simulink model "speedgoat_target_model_2021b"  (R2021b)
settings: Solver=FixedStepAuto  StartTime=0.0  StopTime=inf  RelTol=1e-3
undefined symbols (not defined in the file): DEND_B, DEND_T, DiscIntNeverNeededParam, NUMD_B, NUMD_T, ts
libraries: slrealtimeutilitieslib x7, slrealtimeiplib x7, simulink x5, drivingvehiclecontroller x2, mpcadaslib x1
settings Model: Creator=Buckeye Autodrive  LastModifiedBy=Buckeye Autodrive
settings SolverCC: ConcurrentTasks=on  PositivePriorityOrder=on  AutoInsertRateTranBlk=on
settings OptimizationCC: BlockReduction=off  OptimizeBlockIOStorage=off
settings DebuggingCC: TasksWithSamePriorityMsg=none  UnconnectedInputMsg=none  UnconnectedOutputMsg=none  UnconnectedLineMsg=none
settings HardwareCC: ProdBitPerLong=64  ProdLongLongMode=on  ProdHWDeviceType=Intel->x86-64 (Linux 64)
settings ModelReferenceCC: EnableRefExpFcnMdlSchedulingChecks=off
settings RTWCC: Description=Simulink Real-Time  SystemTargetFile=slrealtime.tlc  TemplateMakefile=slrealtime_default_tmf  Toolchain=Simulink Real-Time Toolchain  BuildConfiguration=Faster Runs  CodeExecutionProfiling=on  TargetLang=C++  DLArmComputeVersion=20.02.1

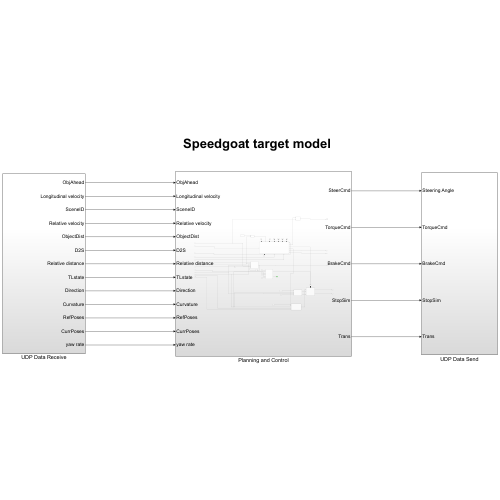
[thumbnail: Simulink's stored preview of the top-level diagram]
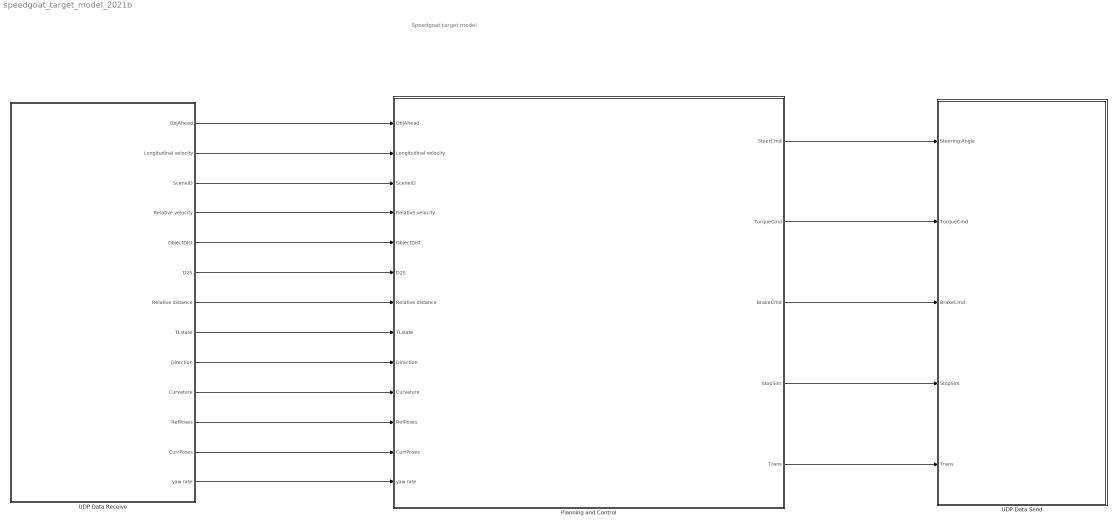
== system speedgoat_target_model_2021b ==
  note: Speedgoat target model
  Planning and Control : Subsystem
  UDP Data Receive : Subsystem
  UDP Data Send : Subsystem
  wires:
  Planning and Control/1(SteerCmd) -> UDP Data Send/1(Steering Angle)
  Planning and Control/2(TorqueCmd) -> UDP Data Send/2(TorqueCmd)
  Planning and Control/3(BrakeCmd) -> UDP Data Send/3(BrakeCmd)
  Planning and Control/4(StopSim) -> UDP Data Send/4(StopSim)
  Planning and Control/5(Trans) -> UDP Data Send/5(Trans)
  UDP Data Receive/1(ObjAhead) -> Planning and Control/1(ObjAhead)
  UDP Data Receive/2(Longitudinal velocity) -> Planning and Control/2(Longitudinal velocity)
  UDP Data Receive/3(SceneID) -> Planning and Control/3(SceneID)
  UDP Data Receive/4(Relative velocity) -> Planning and Control/4(Relative velocity)
  UDP Data Receive/5(ObjectDist) -> Planning and Control/5(ObjectDist)
  UDP Data Receive/6(D2S) -> Planning and Control/6(D2S)
  UDP Data Receive/7(Relative distance) -> Planning and Control/7(Relative distance)
  UDP Data Receive/8(TLstate) -> Planning and Control/8(TLstate)
  UDP Data Receive/9(Direction) -> Planning and Control/9(Direction)
  UDP Data Receive/10(Curvature) -> Planning and Control/10(Curvature)
  UDP Data Receive/11(RefPoses) -> Planning and Control/11(RefPoses)
  UDP Data Receive/12(CurrPoses) -> Planning and Control/12(CurrPoses)
  UDP Data Receive/13(yaw rate) -> Planning and Control/13(yaw rate)

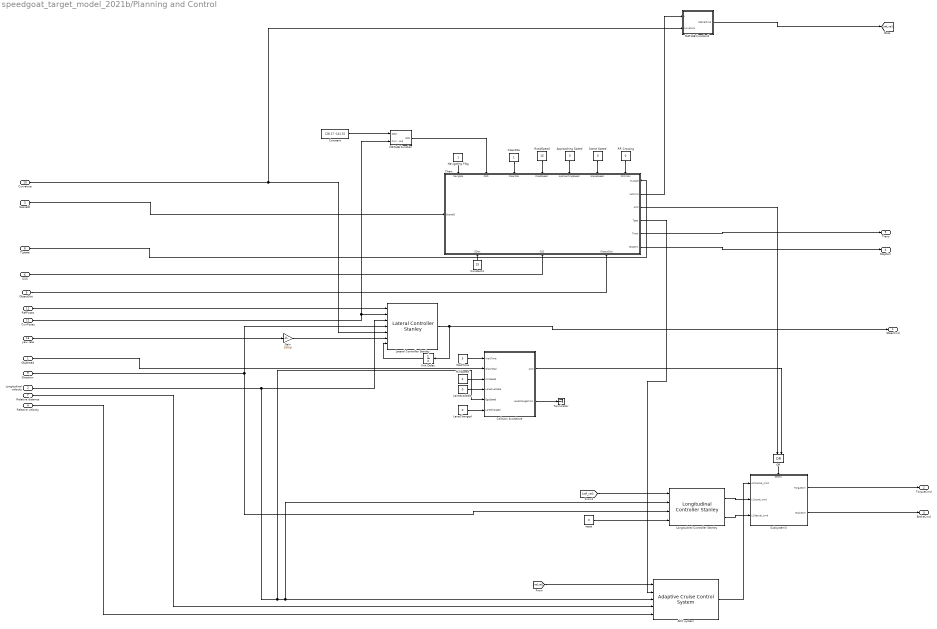
== system speedgoat_target_model_2021b/Planning and Control ==
  ObjAhead : Inport
  Longitudinal velocity : Inport  Port=2
  SceneID : Inport  Port=3
  Relative velocity : Inport  Port=4
  ObjectDist : Inport  Port=5
  D2S : Inport  Port=6
  Relative distance : Inport  Port=7
  TLstate : Inport  Port=8
  Direction : Inport  Port=9
  Curvature : Inport  Port=10
  RefPoses : Inport  Port=11
  CurrPoses : Inport  Port=12
  yaw rate : Inport  Port=13
  ACC system : mpcadaslib/Adaptive Cruise Control System  EgoModel=tf(1,[0.5,1,0])  InitialEgoVelocity=0  DefaultSpacing=4.685  MaxVelocity=50  MinAcceleration=-40  amin_ext=off  MaxAcceleration=40  amax_ext=off  Ts=1  PredictionHorizon=10  ControllerBehavior=1.0  suboptimal=off  maxiter=10  datatypeopt=double  optmode=off  trackmode=off
  Approaching Speed : Constant  Value=5
  Chart : Stateflow chart  TreatAsAtomicUnit=on
      settings: PortSchema="{\"entries\":[{\"content\":{\"sides\":[{\"content\":{\"connectorIds\":[\"In12\"]},\"type\":\"ConnectorPlacement.EquallySpacedRectSide\",\"uuid\":\"81aca70f-0947-49fb-b60a-be241e44193b\"},{\"content\":{\"connectorIds\":[\"In1\",\"Out1\",\"Out2\",\"Out3\",\"Out4\",\"Out5\"],\"side\":\"RIGHT\"},\"type\":\"ConnectorPlacement.EquallySpacedRectSide\",\"uuid\":\"e7b9645e-3711-4964-ac9b-0199dd335e99\"},{\"content\":{\"connectorIds\":[\"In8\",\"In9\",\"In10\",\"In11\",\"In2\",\"In4\",\"In6\"],\"side\":\"TOP\"},\"type\":\"ConnectorPlacement.EquallySpacedRectSide\",\"uuid\":\"6876f024-944b-4540-9404-d68f37763657\"},{\"content\":{\"connectorIds\":[\"In5\",\"In7\",\"In3\"],\"side\":\"BOTTOM\"},\"type\":\"ConnectorPlacement.EquallySpacedRectSide\",\"uuid\":\"44acab73-cdde-4edf-95df-27422644ccab\"}]},\"type\":\"ConnectorPlacement.EquallySpacedConnector\",\"uuid\":\"d2c31c01-e447-43db-8d2b-8b98a0ca291a\"}],\"packageUris\":[\"http://schema.mathworks.com/mf0/Connector/R2020b\"],\"version\":\"1.0\"}"
  Clear2Go : Constant
  Collision Avoidance : Stateflow chart  TreatAsAtomicUnit=on
  Constant : Constant  Value=[28.17 -141.5]
  Constant1 : Constant  Value=25
  Gain : Gain  Gain=180/pi
  LaneAvailable : Constant  Value=0
  LaneChanged : Constant  Value=0
  Lateral Controller Stanley : drivingvehiclecontroller/Lateral Controller Stanley  ModelType=Dynamic bicycle model  PositionGainF=2.5  PositionGainR=2.5  YawRateGain=0.2  DelayGain=0.2  VehicleMass=1853  Lf=1.3425  Lr=1.3425  TireStiffness=5e3  Wheelbase=3  MaxSteeringAngle=80
      settings: SourceProductBaseCode=DR
  Longitudinal Controller Stanley : drivingvehiclecontroller/Longitudinal Controller Stanley  Kp=10  Ki=0.1  SampleTime=1  MaxAcceleration=40  MaxDeceleration=40
      settings: SourceProductBaseCode=DR
  MATLAB Function : MATLAB Function  TreatAsAtomicUnit=on
  MATLAB Function2 : MATLAB Function  TreatAsAtomicUnit=on
  MinSpeed : Constant  Value=2
  Navigating Flag : Constant
  OR : Logic  Operator=OR  IconShape=distinctive  AllPortsSameDT=off  OutDataTypeStr=fixdt(1,16)
  RR Crossing : Constant  Value=0
  RoadSpeed : Constant  Value=15
  Scene Speed : Constant  Value=5
  Subsystem3 : Subsystem
      settings: PortSchema="{\"entries\":[{\"content\":{\"sides\":[{\"content\":{\"connectorIds\":[\"In1\",\"In2\",\"In3\"]},\"type\":\"ConnectorPlacement.EquallySpacedRectSide\",\"uuid\":\"a23b1a10-3bcb-40a0-900c-c9a3f160b173\"},{\"content\":{\"connectorIds\":[\"Out1\",\"Out2\"],\"side\":\"RIGHT\"},\"type\":\"ConnectorPlacement.EquallySpacedRectSide\",\"uuid\":\"88840b66-912f-4184-aeec-297642319416\"},{\"content\":{\"connectorIds\":[\"In4\"],\"side\":\"TOP\"},\"type\":\"ConnectorPlacement.EquallySpacedRectSide\",\"uuid\":\"37a03ca9-b065-473e-b290-3b07703c6005\"}]},\"type\":\"ConnectorPlacement.EquallySpacedConnector\",\"uuid\":\"5bfc7c71-8f7a-4cba-a168-7eeca22a2fcb\"}],\"packageUris\":[\"http://schema.mathworks.com/mf0/Connector/R2020b\"],\"version\":\"1.0\"}"
  Terminator : Terminator
  Unit Delay : UnitDelay  SampleTime=-1  HasFrameUpgradeWarning=on
  WaitTime : Constant  Value=3
  reset : Constant  Value=0
  SteerCmd : Outport
  TorqueCmd : Outport  Port=2
  BrakeCmd : Outport  Port=3
  StopSim : Outport  Port=4
  Trans : Outport  Port=5
  wires:
  TLstate/1 -> Chart/1(TLstate)
  Chart/3(Tgap) -> ACC system/2
  Collision Avoidance/2(LaneChangeCmd) -> Terminator/1
  Navigating Flag/1 -> Chart/8(Navigate)
  Longitudinal velocity/1 -> Collision Avoidance/5(EgoSpeed), Longitudinal Controller Stanley/2, ACC system/3, Lateral Controller Stanley/3
  MinSpeed/1 -> Collision Avoidance/3(MinSpeed)
  RefPoses/1 -> Lateral Controller Stanley/1
  yaw rate/1 -> Gain/1
  Lateral Controller Stanley/1 -> Unit Delay/1, SteerCmd/1
  Constant1/1 -> Chart/5(SDist)
  ACC system/1 -> Subsystem3/1(ACCaccel_cmd)
  Scene Speed/1 -> Chart/4(SceneSpeed)
  Curvature/1 -> Lateral Controller Stanley/5, MATLAB Function2/2(curvature)
  Chart/2(ACC) -> OR/1
  [ref_vel] -> ACC system/1
  Collision Avoidance/1(ACC) -> OR/2
  [ref_vel] -> Longitudinal Controller Stanley/1
  Subsystem3/1(TorgueCm) -> TorqueCmd/1
  ObjAhead/1 -> Collision Avoidance/2(ObjAhead)
  SceneID/1 -> Chart/12(SceneID)
  Direction/1 -> Longitudinal Controller Stanley/3, Lateral Controller Stanley/4
  MATLAB Function/1(D2D) -> Chart/9(D2D)
  Constant/1 -> MATLAB Function/1(Dest)
  RoadSpeed/1 -> Chart/11(RoadSpeed)
  Longitudinal Controller Stanley/1 -> Subsystem3/2(LCaccel_cmd)
  reset/1 -> Longitudinal Controller Stanley/4
  CurrPoses/1 -> MATLAB Function/2(CurrentPose), Lateral Controller Stanley/2
  LaneChanged/1 -> Collision Avoidance/6(LaneChanged)
  Clear2Go/1 -> Chart/10(Clear2Go)
  Longitudinal Controller Stanley/2 -> Subsystem3/3(LCdeccel_cmd)
  RR Crossing/1 -> Chart/6(RRCross)
  Chart/1(VelCmd) -> MATLAB Function2/1(v)
  ObjectDist/1 -> Chart/3(ObjectDist)
  WaitTime/1 -> Collision Avoidance/1(WaitTime)
  Chart/4(Trans) -> Trans/1
  LaneAvailable/1 -> Collision Avoidance/4(LaneAvailable)
  Chart/5(StopSim) -> StopSim/1
  Approaching Speed/1 -> Chart/2(ApproachingSpeed)
  OR/1 -> Subsystem3/4(Select)
  Relative distance/1 -> ACC system/4
  Subsystem3/2(BrakeCm) -> BrakeCmd/1
  Relative velocity/1 -> ACC system/5
  D2S/1 -> Chart/7(D2S)
  MATLAB Function2/1(RefVelCmd) -> [ref_vel]
  Gain/1 -> Lateral Controller Stanley/6
  Unit Delay/1 -> Lateral Controller Stanley/7

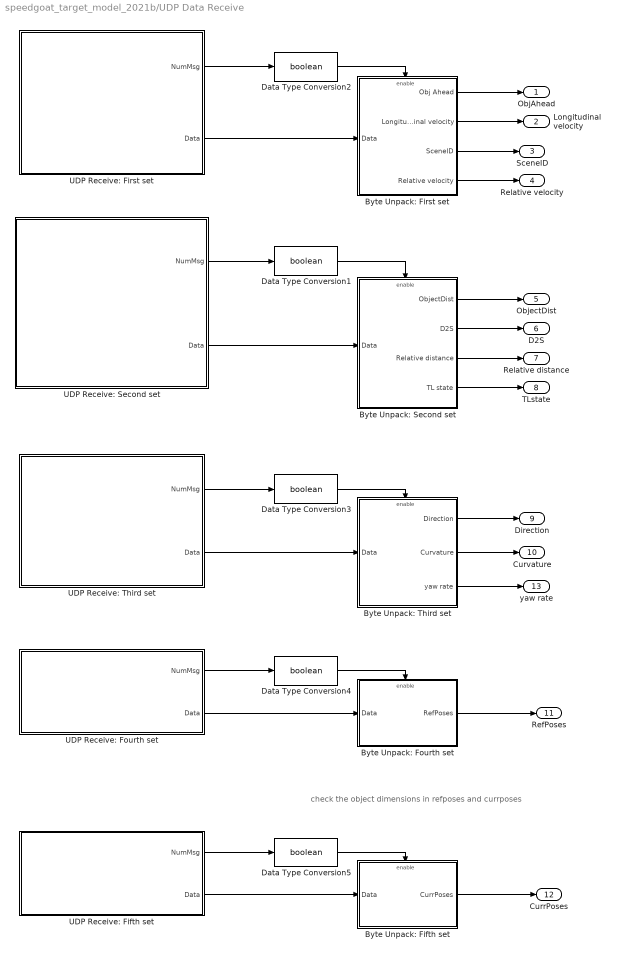
== system speedgoat_target_model_2021b/UDP Data Receive ==
  note: check the object dimensions in refposes and currposes
  Byte Unpack: Fifth set : Subsystem
  Byte Unpack: First set : Subsystem
  Byte Unpack: Fourth set : Subsystem
  Byte Unpack: Second set : Subsystem
  Byte Unpack: Third set : Subsystem
  Data Type Conversion{1..5} (5 alike) : DataTypeConversion  OutDataTypeStr=boolean
  UDP Receive: Fifth set : Subsystem
  UDP Receive: First set : Subsystem
  UDP Receive: Fourth set : Subsystem
  UDP Receive: Second set : Subsystem
  UDP Receive: Third set : Subsystem
  ObjAhead : Outport
  Longitudinal velocity : Outport  Port=2
  SceneID : Outport  Port=3
  Relative velocity : Outport  Port=4
  ObjectDist : Outport  Port=5
  D2S : Outport  Port=6
  Relative distance : Outport  Port=7
  TLstate : Outport  Port=8
  Direction : Outport  Port=9
  Curvature : Outport  Port=10
  RefPoses : Outport  Port=11
  CurrPoses : Outport  Port=12
  yaw rate : Outport  Port=13
  wires:
  UDP Receive: First set/1(NumMsg) -> Data Type Conversion2/1
  Data Type Conversion2/1 -> Byte Unpack: First set/Enable
  UDP Receive: First set/2(Data) -> Byte Unpack: First set/1(Data)
  UDP Receive: Second set/2(Data) -> Byte Unpack: Second set/1(Data)
  Data Type Conversion1/1 -> Byte Unpack: Second set/Enable
  UDP Receive: Second set/1(NumMsg) -> Data Type Conversion1/1
  UDP Receive: Third set/1(NumMsg) -> Data Type Conversion3/1
  Data Type Conversion3/1 -> Byte Unpack: Third set/Enable
  UDP Receive: Third set/2(Data) -> Byte Unpack: Third set/1(Data)
  UDP Receive: Fifth set/2(Data) -> Byte Unpack: Fifth set/1(Data)
  Data Type Conversion5/1 -> Byte Unpack: Fifth set/Enable
  UDP Receive: Fifth set/1(NumMsg) -> Data Type Conversion5/1
  UDP Receive: Fourth set/1(NumMsg) -> Data Type Conversion4/1
  Data Type Conversion4/1 -> Byte Unpack: Fourth set/Enable
  UDP Receive: Fourth set/2(Data) -> Byte Unpack: Fourth set/1(Data)
  Byte Unpack: First set/1(Obj Ahead) -> ObjAhead/1
  Byte Unpack: First set/2(Longitudinal velocity) -> Longitudinal velocity/1
  Byte Unpack: First set/3(SceneID) -> SceneID/1
  Byte Unpack: First set/4(Relative velocity) -> Relative velocity/1
  Byte Unpack: Second set/1(ObjectDist) -> ObjectDist/1
  Byte Unpack: Second set/2(D2S) -> D2S/1
  Byte Unpack: Second set/3(Relative distance) -> Relative distance/1
  Byte Unpack: Second set/4(TL state) -> TLstate/1
  Byte Unpack: Fourth set/1(RefPoses) -> RefPoses/1
  Byte Unpack: Fifth set/1(CurrPoses) -> CurrPoses/1
  Byte Unpack: Third set/1(Direction) -> Direction/1
  Byte Unpack: Third set/2(Curvature) -> Curvature/1
  Byte Unpack: Third set/3(yaw rate) -> yaw rate/1

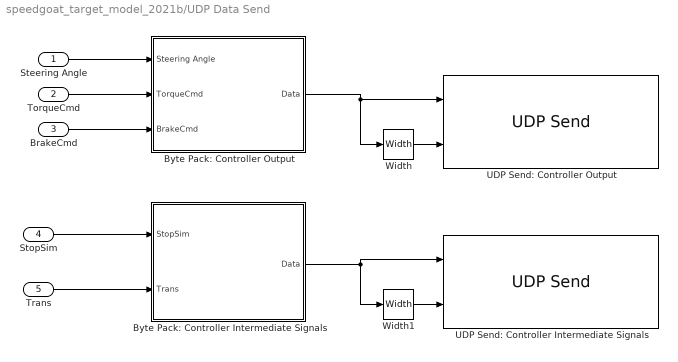
== system speedgoat_target_model_2021b/UDP Data Send ==
  Steering Angle : Inport
  TorqueCmd : Inport  Port=2
  BrakeCmd : Inport  Port=3
  StopSim : Inport  Port=4
  Trans : Inport  Port=5
  Byte Pack: Controller Intermediate Signals : Subsystem
  Byte Pack: Controller Output : Subsystem
  UDP Send: Controller Intermediate Signals : slrealtimeiplib/UDP Send  useHostTargetConn=on  toAddress=192.168.7.1  toPort=8017  sampleTime=0.1  ipAddress=192.168.7.2  localPort=-1
      settings: SourceProductBaseCode=XP
  UDP Send: Controller Output : slrealtimeiplib/UDP Send  useHostTargetConn=on  toAddress=192.168.7.1  toPort=8016  sampleTime=0.1  ipAddress=192.168.7.2  localPort=-1
      settings: SourceProductBaseCode=XP
  Width : Width
  Width1 : Width
  wires:
  Width1/1 -> UDP Send: Controller Intermediate Signals/2
  Width/1 -> UDP Send: Controller Output/2
  Byte Pack: Controller Output/1(Data) -> Width/1, UDP Send: Controller Output/1
  Steering Angle/1 -> Byte Pack: Controller Output/1(Steering Angle)
  TorqueCmd/1 -> Byte Pack: Controller Output/2(TorqueCmd)
  Byte Pack: Controller Intermediate Signals/1(Data) -> UDP Send: Controller Intermediate Signals/1, Width1/1
  StopSim/1 -> Byte Pack: Controller Intermediate Signals/1(StopSim)
  Trans/1 -> Byte Pack: Controller Intermediate Signals/2(Trans)
  BrakeCmd/1 -> Byte Pack: Controller Output/3(BrakeCmd)

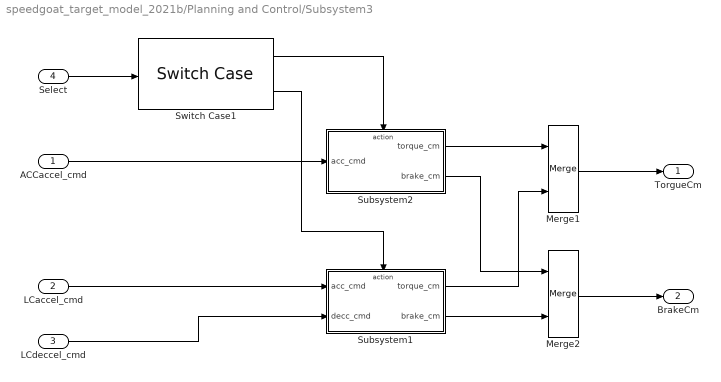
== system speedgoat_target_model_2021b/Planning and Control/Subsystem3 ==
  ACCaccel_cmd : Inport
  LCaccel_cmd : Inport  Port=2
  LCdeccel_cmd : Inport  Port=3
  Select : Inport  Port=4
  Merge1 : Merge
  Merge2 : Merge
  Subsystem1 : Subsystem
  Subsystem2 : Subsystem
  Switch Case1 : SwitchCase  CaseConditions={1, 0}  ShowDefaultCase=off
  TorgueCm : Outport
  BrakeCm : Outport  Port=2
  wires:
  LCdeccel_cmd/1 -> Subsystem1/2(decc_cmd)
  Subsystem1/2(brake_cm) -> Merge2/2
  Subsystem1/1(torque_cm) -> Merge1/2
  Subsystem2/2(brake_cm) -> Merge2/1
  Switch Case1/1 -> Subsystem2/Action
  Switch Case1/2 -> Subsystem1/Action
  Subsystem2/1(torque_cm) -> Merge1/1
  LCaccel_cmd/1 -> Subsystem1/1(acc_cmd)
  Merge2/1 -> BrakeCm/1
  ACCaccel_cmd/1 -> Subsystem2/1(acc_cmd)
  Merge1/1 -> TorgueCm/1
  Select/1 -> Switch Case1/1

== system speedgoat_target_model_2021b/UDP Data Receive/Byte Unpack: Fifth set ==
  Data : Inport
  Enable : EnablePort
  Byte Unpacking 1 : slrealtimeutilitieslib/Byte Unpacking  MaskUnpackedDataTypes={'double'}  MaskUnpackedDataSizes={[3]}  MaskAlignment=1
      settings: SourceProductBaseCode=XP
  CurrPoses : Outport
  wires:
  Data/1 -> Byte Unpacking 1/1
  Byte Unpacking 1/1 -> CurrPoses/1  "CurrPoses"

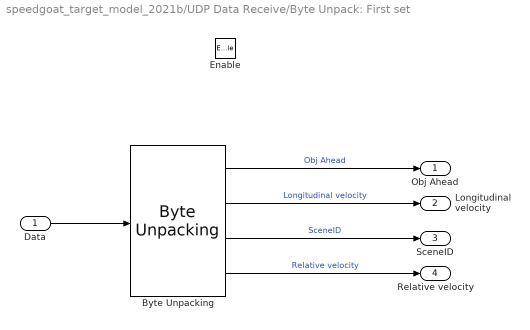
== system speedgoat_target_model_2021b/UDP Data Receive/Byte Unpack: First set ==
  Data : Inport
  Enable : EnablePort
  "Byte Unpacking " : slrealtimeutilitieslib/Byte Unpacking  MaskUnpackedDataTypes={'double', 'double', 'double', 'double'}  MaskUnpackedDataSizes={[1], [1], [1], [1]}  MaskAlignment=1
      settings: SourceProductBaseCode=XP
  Obj Ahead : Outport
  Longitudinal velocity : Outport  Port=2
  SceneID : Outport  Port=3
  Relative velocity : Outport  Port=4
  wires:
  Data/1 -> "Byte Unpacking "/1
  "Byte Unpacking "/1 -> Obj Ahead/1  "Obj Ahead"
  "Byte Unpacking "/2 -> Longitudinal velocity/1  "Longitudinal velocity"
  "Byte Unpacking "/3 -> SceneID/1  "SceneID"
  "Byte Unpacking "/4 -> Relative velocity/1  "Relative velocity"

== system speedgoat_target_model_2021b/UDP Data Receive/Byte Unpack: Fourth set ==
  Data : Inport
  Enable : EnablePort
  "Byte Unpacking " : slrealtimeutilitieslib/Byte Unpacking  MaskUnpackedDataTypes={'double'}  MaskUnpackedDataSizes={[3]}  MaskAlignment=1
      settings: SourceProductBaseCode=XP
  RefPoses : Outport
  wires:
  Data/1 -> "Byte Unpacking "/1
  "Byte Unpacking "/1 -> RefPoses/1  "RefPoses"

== system speedgoat_target_model_2021b/UDP Data Receive/Byte Unpack: Second set ==
  Data : Inport
  Enable : EnablePort
  "Byte Unpacking " : slrealtimeutilitieslib/Byte Unpacking  MaskUnpackedDataTypes={'double', 'double', 'double', 'double'}  MaskUnpackedDataSizes={[1], [1], [1], [18,5]}  MaskAlignment=1
      settings: SourceProductBaseCode=XP
  ObjectDist : Outport
  D2S : Outport  Port=2
  Relative distance : Outport  Port=3
  TL state : Outport  Port=4
  wires:
  "Byte Unpacking "/4 -> TL state/1  "TL state"
  "Byte Unpacking "/3 -> Relative distance/1  "Relative distance"
  "Byte Unpacking "/2 -> D2S/1  "D2S"
  "Byte Unpacking "/1 -> ObjectDist/1  "ObjectDist"
  Data/1 -> "Byte Unpacking "/1

== system speedgoat_target_model_2021b/UDP Data Receive/Byte Unpack: Third set ==
  Data : Inport
  Enable : EnablePort
  "Byte Unpacking " : slrealtimeutilitieslib/Byte Unpacking  MaskUnpackedDataTypes={'double', 'double', 'double'}  MaskUnpackedDataSizes={[1], [1], [1]}  MaskAlignment=1
      settings: SourceProductBaseCode=XP
  Direction : Outport
  Curvature : Outport  Port=2
  yaw rate : Outport  Port=3
  wires:
  Data/1 -> "Byte Unpacking "/1
  "Byte Unpacking "/1 -> Direction/1  "Direction"
  "Byte Unpacking "/2 -> Curvature/1  "Curvature"
  "Byte Unpacking "/3 -> yaw rate/1  "yaw rate"

== system speedgoat_target_model_2021b/UDP Data Receive/UDP Receive: Fifth set ==
  Compare To Constant : simulink/Logic and Bit Operations/Compare To Constant  relop===  const=24  OutDataTypeStr=boolean
  Constant : Constant
  Subtract : Sum  Inputs=+-
  UDP Receive2 : slrealtimeiplib/UDP Receive  useHostTargetConn=on  ipAddress=192.168.7.2  localPort=8005  rcvWidth=24  rcvFmAny=off  fmAddress=192.168.7.1  sampleTime=-1
      settings: SourceProductBaseCode=XP
  While Iterator : WhileIterator  WhileBlockType=do-while  ResetStates=reset  ShowIterationPort=on
  NumMsg : Outport
  Data : Outport  Port=2
  wires:
  While Iterator/1 -> Subtract/1
  UDP Receive2/2 -> Compare To Constant/1
  Subtract/1 -> NumMsg/1
  Constant/1 -> Subtract/2
  UDP Receive2/1 -> Data/1
  Compare To Constant/1 -> While Iterator/1

== system speedgoat_target_model_2021b/UDP Data Receive/UDP Receive: First set ==
  Compare To Constant : simulink/Logic and Bit Operations/Compare To Constant  relop===  const=32  OutDataTypeStr=boolean
  Constant : Constant
  Subtract : Sum  Inputs=+-
  UDP Receive2 : slrealtimeiplib/UDP Receive  useHostTargetConn=on  ipAddress=192.168.7.2  localPort=8001  rcvWidth=32  rcvFmAny=off  fmAddress=192.168.7.1  sampleTime=-1
      settings: SourceProductBaseCode=XP
  While Iterator : WhileIterator  WhileBlockType=do-while  ResetStates=reset  ShowIterationPort=on
  NumMsg : Outport
  Data : Outport  Port=2
  wires:
  Compare To Constant/1 -> While Iterator/1
  UDP Receive2/1 -> Data/1
  Constant/1 -> Subtract/2
  Subtract/1 -> NumMsg/1
  UDP Receive2/2 -> Compare To Constant/1
  While Iterator/1 -> Subtract/1

== system speedgoat_target_model_2021b/UDP Data Receive/UDP Receive: Fourth set ==
  Compare To Constant : simulink/Logic and Bit Operations/Compare To Constant  relop===  const=24  OutDataTypeStr=boolean
  Constant : Constant
  Subtract : Sum  Inputs=+-
  UDP Receive2 : slrealtimeiplib/UDP Receive  useHostTargetConn=on  ipAddress=192.168.7.2  localPort=8004  rcvWidth=24  rcvFmAny=off  fmAddress=192.168.7.1  sampleTime=-1
      settings: SourceProductBaseCode=XP
  While Iterator : WhileIterator  WhileBlockType=do-while  ResetStates=reset  ShowIterationPort=on
  NumMsg : Outport
  Data : Outport  Port=2
  wires:
  Compare To Constant/1 -> While Iterator/1
  UDP Receive2/1 -> Data/1
  Constant/1 -> Subtract/2
  Subtract/1 -> NumMsg/1
  UDP Receive2/2 -> Compare To Constant/1
  While Iterator/1 -> Subtract/1

== system speedgoat_target_model_2021b/UDP Data Receive/UDP Receive: Second set ==
  Compare To Constant : simulink/Logic and Bit Operations/Compare To Constant  relop===  const=744  OutDataTypeStr=boolean
  Constant : Constant
  Subtract : Sum  Inputs=+-
  UDP Receive2 : slrealtimeiplib/UDP Receive  useHostTargetConn=on  ipAddress=192.168.7.2  localPort=8002  rcvWidth=744  rcvFmAny=off  fmAddress=192.168.7.1  sampleTime=-1
      settings: SourceProductBaseCode=XP
  While Iterator : WhileIterator  WhileBlockType=do-while  ResetStates=reset  ShowIterationPort=on
  NumMsg : Outport
  Data : Outport  Port=2
  wires:
  While Iterator/1 -> Subtract/1
  UDP Receive2/2 -> Compare To Constant/1
  Subtract/1 -> NumMsg/1
  Constant/1 -> Subtract/2
  UDP Receive2/1 -> Data/1
  Compare To Constant/1 -> While Iterator/1

== system speedgoat_target_model_2021b/UDP Data Receive/UDP Receive: Third set ==
  Compare To Constant : simulink/Logic and Bit Operations/Compare To Constant  relop===  const=24  OutDataTypeStr=boolean
  Constant : Constant
  Subtract : Sum  Inputs=+-
  UDP Receive2 : slrealtimeiplib/UDP Receive  useHostTargetConn=on  ipAddress=192.168.7.2  localPort=8003  rcvWidth=24  rcvFmAny=off  fmAddress=192.168.7.1  sampleTime=-1
      settings: SourceProductBaseCode=XP
  While Iterator : WhileIterator  WhileBlockType=do-while  ResetStates=reset  ShowIterationPort=on
  NumMsg : Outport
  Data : Outport  Port=2
  wires:
  Compare To Constant/1 -> While Iterator/1
  UDP Receive2/1 -> Data/1
  Constant/1 -> Subtract/2
  Subtract/1 -> NumMsg/1
  UDP Receive2/2 -> Compare To Constant/1
  While Iterator/1 -> Subtract/1

== system speedgoat_target_model_2021b/UDP Data Send/Byte Pack: Controller Intermediate Signals ==
  StopSim : Inport
  Trans : Inport  Port=2
  Byte Packing1 : slrealtimeutilitieslib/Byte Packing  MaskPackedDataType=uint8  MaskUnpackedDataTypes={'double', 'double'}  MaskAlignment=1
  Data : Outport
  wires:
  Byte Packing1/1 -> Data/1
  StopSim/1 -> Byte Packing1/1
  Trans/1 -> Byte Packing1/2

== system speedgoat_target_model_2021b/UDP Data Send/Byte Pack: Controller Output ==
  Steering Angle : Inport
  TorqueCmd : Inport  Port=2
  BrakeCmd : Inport  Port=3
  Byte Packing : slrealtimeutilitieslib/Byte Packing  MaskPackedDataType=uint8  MaskUnpackedDataTypes={'double', 'double','double'}  MaskAlignment=1
  Data : Outport
  wires:
  TorqueCmd/1 -> Byte Packing/2
  Byte Packing/1 -> Data/1
  Steering Angle/1 -> Byte Packing/1
  BrakeCmd/1 -> Byte Packing/3

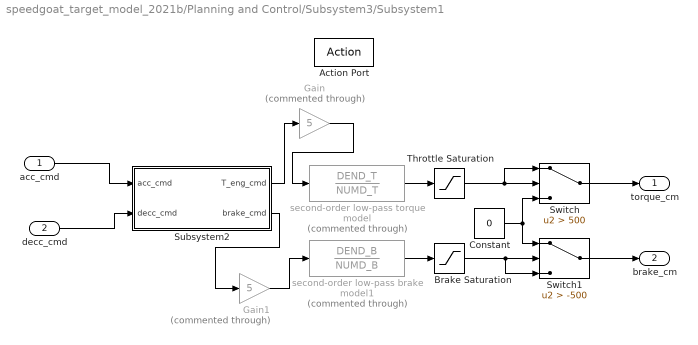
== system speedgoat_target_model_2021b/Planning and Control/Subsystem3/Subsystem1 ==
  acc_cmd : Inport
  decc_cmd : Inport  Port=2
  Action Port : ActionPort  ActionPortLabel=case [ 0 ]:
  Brake Saturation : Saturate  UpperLimit=0  LowerLimit=-65534
  Constant : Constant  Value=0
  Gain : Gain  Commented=through  Gain=5
  Gain1 : Gain  Commented=through  Gain=5
  Subsystem2 : Subsystem
  Switch : Switch  Criteria=u2 > Threshold  Threshold=500
  Switch1 : Switch  Criteria=u2 > Threshold  Threshold=-500
  Throttle Saturation : Saturate  UpperLimit=22534  LowerLimit=-22534
  second-order low-pass brake model1 : DiscreteTransferFcn  Commented=through  Numerator=DEND_B  Denominator=NUMD_B  SampleTime=ts
  second-order low-pass torque model : DiscreteTransferFcn  Commented=through  Numerator=DEND_T  Denominator=NUMD_T  SampleTime=ts
  torque_cm : Outport
  brake_cm : Outport  Port=2
  wires:
  acc_cmd/1 -> Subsystem2/1(acc_cmd)
  Throttle Saturation/1 -> Switch/2, Switch/1
  decc_cmd/1 -> Subsystem2/2(decc_cmd)
  Subsystem2/1(T_eng_cmd) -> Gain/1
  Brake Saturation/1 -> Switch1/2, Switch1/3
  Gain/1 -> second-order low-pass torque model/1
  Gain1/1 -> second-order low-pass brake model1/1
  Subsystem2/2(brake_cmd) -> Gain1/1
  Constant/1 -> Switch/3, Switch1/1
  Switch1/1 -> brake_cm/1
  Switch/1 -> torque_cm/1
  second-order low-pass torque model/1 -> Throttle Saturation/1
  second-order low-pass brake model1/1 -> Brake Saturation/1

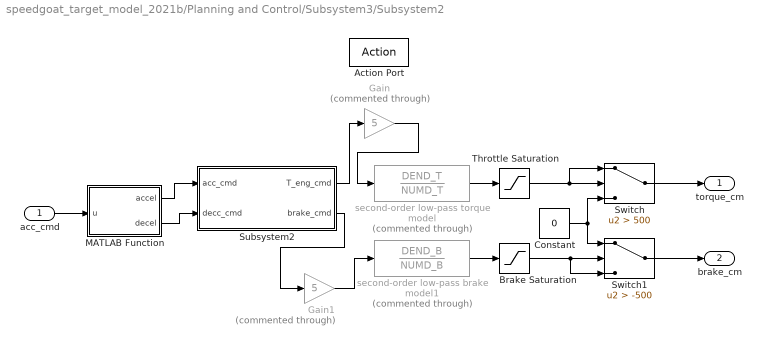
== system speedgoat_target_model_2021b/Planning and Control/Subsystem3/Subsystem2 ==
  acc_cmd : Inport
  Action Port : ActionPort  ActionPortLabel=case [ 1 ]:
  Brake Saturation : Saturate  UpperLimit=0  LowerLimit=-65534
  Constant : Constant  Value=0
  Gain : Gain  Commented=through  Gain=5
  Gain1 : Gain  Commented=through  Gain=5
  MATLAB Function : MATLAB Function  TreatAsAtomicUnit=on
  Subsystem2 : Subsystem
  Switch : Switch  Criteria=u2 > Threshold  Threshold=500
  Switch1 : Switch  Criteria=u2 > Threshold  Threshold=-500
  Throttle Saturation : Saturate  UpperLimit=22534  LowerLimit=-22534
  second-order low-pass brake model1 : DiscreteTransferFcn  Commented=through  Numerator=DEND_B  Denominator=NUMD_B  SampleTime=ts
  second-order low-pass torque model : DiscreteTransferFcn  Commented=through  Numerator=DEND_T  Denominator=NUMD_T  SampleTime=ts
  torque_cm : Outport
  brake_cm : Outport  Port=2
  wires:
  second-order low-pass brake model1/1 -> Brake Saturation/1
  second-order low-pass torque model/1 -> Throttle Saturation/1
  Throttle Saturation/1 -> Switch/2, Switch/1
  Switch/1 -> torque_cm/1
  Brake Saturation/1 -> Switch1/2, Switch1/3
  Switch1/1 -> brake_cm/1
  Constant/1 -> Switch/3, Switch1/1
  acc_cmd/1 -> MATLAB Function/1(u)
  MATLAB Function/1(accel) -> Subsystem2/1(acc_cmd)
  MATLAB Function/2(decel) -> Subsystem2/2(decc_cmd)
  Subsystem2/1(T_eng_cmd) -> Gain/1
  Gain/1 -> second-order low-pass torque model/1
  Gain1/1 -> second-order low-pass brake model1/1
  Subsystem2/2(brake_cmd) -> Gain1/1

== system speedgoat_target_model_2021b/Planning and Control/Subsystem3/Subsystem1/Subsystem2 ==
  acc_cmd : Inport
  decc_cmd : Inport  Port=2
  Subsystem : Subsystem
  Subsystem1 : Subsystem
  T_eng_cmd : Outport
  brake_cmd : Outport  Port=2
  wires:
  acc_cmd/1 -> Subsystem/1(acc_cmd)
  Subsystem/1(T_eng_cmd) -> T_eng_cmd/1
  decc_cmd/1 -> Subsystem1/1(decc_cmd)
  Subsystem1/1(T_brake_cmd) -> brake_cmd/1

== system speedgoat_target_model_2021b/Planning and Control/Subsystem3/Subsystem2/Subsystem2 ==
  acc_cmd : Inport
  decc_cmd : Inport  Port=2
  Subsystem : Subsystem
  Subsystem1 : Subsystem
  T_eng_cmd : Outport
  brake_cmd : Outport  Port=2
  wires:
  acc_cmd/1 -> Subsystem/1(acc_cmd)
  Subsystem/1(T_eng_cmd) -> T_eng_cmd/1
  decc_cmd/1 -> Subsystem1/1(decc_cmd)
  Subsystem1/1(T_brake_cmd) -> brake_cmd/1

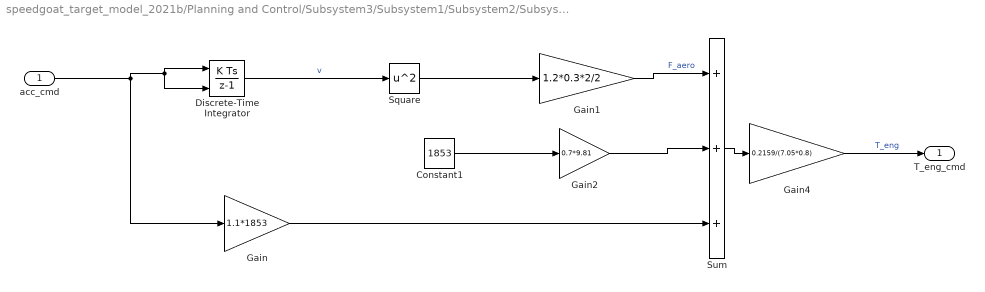
== system speedgoat_target_model_2021b/Planning and Control/Subsystem3/Subsystem1/Subsystem2/Subsystem ==
  acc_cmd : Inport
  Constant1 : Constant  Value=1853
  Discrete-Time Integrator : DiscreteIntegrator  ExternalReset=falling  SampleTime=-1  ICPrevOutput=DiscIntNeverNeededParam  ICPrevScaledInput=DiscIntNeverNeededParam
  Gain : Gain  Gain=1.1*1853
  Gain1 : Gain  Gain=1.2*0.3*2/2
  Gain2 : Gain  Gain=0.7*9.81
  Gain4 : Gain  Gain=0.2159/(7.05*0.8)
  Square : Math  Operator=square  SaturateOnIntegerOverflow=on
  Sum : Sum  Inputs=+++
  T_eng_cmd : Outport
  wires:
  Constant1/1 -> Gain2/1
  Gain/1 -> Sum/3
  Sum/1 -> Gain4/1
  acc_cmd/1 -> Gain/1, Discrete-Time Integrator/1, Discrete-Time Integrator/2
  Gain2/1 -> Sum/2
  Gain1/1 -> Sum/1  "F_aero"
  Gain4/1 -> T_eng_cmd/1  "T_eng"
  Discrete-Time Integrator/1 -> Square/1  "v"
  Square/1 -> Gain1/1

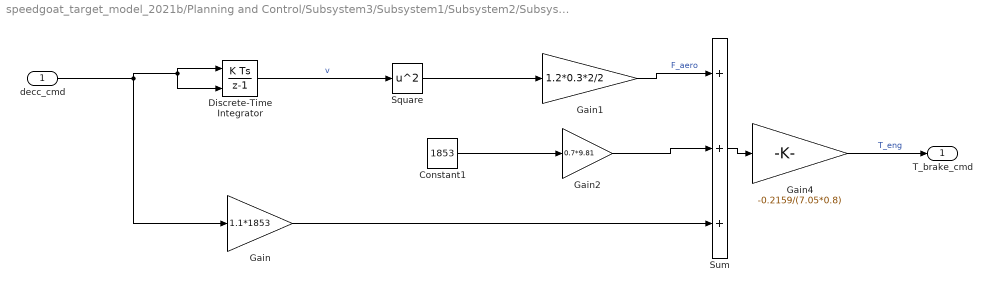
== system speedgoat_target_model_2021b/Planning and Control/Subsystem3/Subsystem1/Subsystem2/Subsystem1 ==
  decc_cmd : Inport
  Constant1 : Constant  Value=1853
  Discrete-Time Integrator : DiscreteIntegrator  ExternalReset=falling  SampleTime=-1  ICPrevOutput=DiscIntNeverNeededParam  ICPrevScaledInput=DiscIntNeverNeededParam
  Gain : Gain  Gain=1.1*1853
  Gain1 : Gain  Gain=1.2*0.3*2/2
  Gain2 : Gain  Gain=0.7*9.81
  Gain4 : Gain  Gain=-0.2159/(7.05*0.8)
  Square : Math  Operator=square  SaturateOnIntegerOverflow=on
  Sum : Sum  Inputs=+++
  T_brake_cmd : Outport
  wires:
  Square/1 -> Gain1/1
  Discrete-Time Integrator/1 -> Square/1  "v"
  Gain4/1 -> T_brake_cmd/1  "T_eng"
  Gain1/1 -> Sum/1  "F_aero"
  Gain2/1 -> Sum/2
  decc_cmd/1 -> Discrete-Time Integrator/2, Discrete-Time Integrator/1, Gain/1
  Sum/1 -> Gain4/1
  Gain/1 -> Sum/3
  Constant1/1 -> Gain2/1

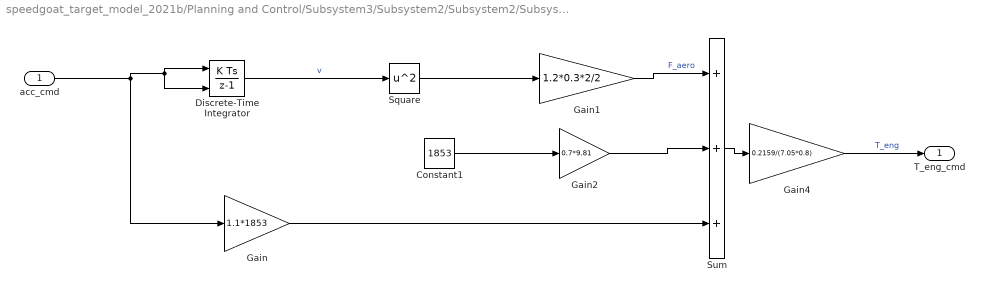
== system speedgoat_target_model_2021b/Planning and Control/Subsystem3/Subsystem2/Subsystem2/Subsystem ==
  acc_cmd : Inport
  Constant1 : Constant  Value=1853
  Discrete-Time Integrator : DiscreteIntegrator  ExternalReset=falling  SampleTime=-1  ICPrevOutput=DiscIntNeverNeededParam  ICPrevScaledInput=DiscIntNeverNeededParam
  Gain : Gain  Gain=1.1*1853
  Gain1 : Gain  Gain=1.2*0.3*2/2
  Gain2 : Gain  Gain=0.7*9.81
  Gain4 : Gain  Gain=0.2159/(7.05*0.8)
  Square : Math  Operator=square  SaturateOnIntegerOverflow=on
  Sum : Sum  Inputs=+++
  T_eng_cmd : Outport
  wires:
  Constant1/1 -> Gain2/1
  Gain/1 -> Sum/3
  Sum/1 -> Gain4/1
  acc_cmd/1 -> Gain/1, Discrete-Time Integrator/1, Discrete-Time Integrator/2
  Gain2/1 -> Sum/2
  Gain1/1 -> Sum/1  "F_aero"
  Gain4/1 -> T_eng_cmd/1  "T_eng"
  Discrete-Time Integrator/1 -> Square/1  "v"
  Square/1 -> Gain1/1

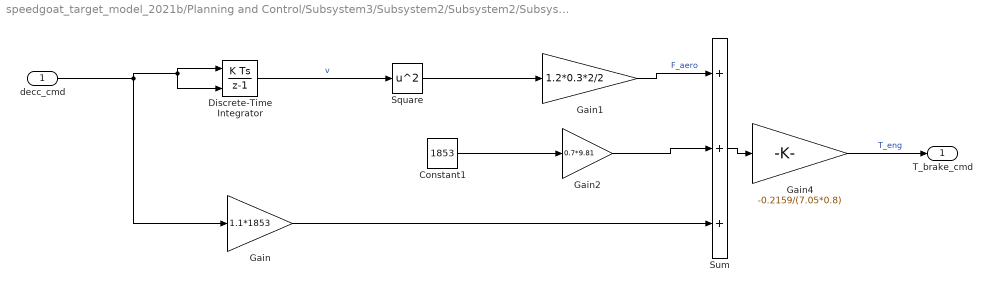
== system speedgoat_target_model_2021b/Planning and Control/Subsystem3/Subsystem2/Subsystem2/Subsystem1 ==
  decc_cmd : Inport
  Constant1 : Constant  Value=1853
  Discrete-Time Integrator : DiscreteIntegrator  ExternalReset=falling  SampleTime=-1  ICPrevOutput=DiscIntNeverNeededParam  ICPrevScaledInput=DiscIntNeverNeededParam
  Gain : Gain  Gain=1.1*1853
  Gain1 : Gain  Gain=1.2*0.3*2/2
  Gain2 : Gain  Gain=0.7*9.81
  Gain4 : Gain  Gain=-0.2159/(7.05*0.8)
  Square : Math  Operator=square  SaturateOnIntegerOverflow=on
  Sum : Sum  Inputs=+++
  T_brake_cmd : Outport
  wires:
  Square/1 -> Gain1/1
  Discrete-Time Integrator/1 -> Square/1  "v"
  Gain4/1 -> T_brake_cmd/1  "T_eng"
  Gain1/1 -> Sum/1  "F_aero"
  Gain2/1 -> Sum/2
  decc_cmd/1 -> Discrete-Time Integrator/2, Discrete-Time Integrator/1, Gain/1
  Sum/1 -> Gain4/1
  Gain/1 -> Sum/3
  Constant1/1 -> Gain2/1

== stateflow chart speedgoat_target_model_2021b/Planning and Control/Collision Avoidance ==
  state Start
    en:
    Stuck = 0;
    ACC = 0;
    LaneChangeCmd = 0;
    %VelCmd = CurrentVelCmd;
  state Follow
    en:
    ACC = 1;
  state LaneChange
    en:
    LaneChangeCmd = 1;
  LaneChange -> Start : [LaneChanged == 1]
  (default) -> Start
  Follow -> LaneChange [order 2] : [LaneAvailable == 1 && Stuck == 1]
  Start -> Follow : [ObjAhead == 1]
  Follow -> Start [order 3] : [ObjAhead == 0]
  Follow -> Follow [order 1] : [(EgoSpeed <= MinSpeed) && after(WaitTime,sec)]{Stuck = 1;}
  data: Stuck local; ACC output; WaitTime input; ObjAhead input; MinSpeed input; LaneAvailable input; EgoSpeed input; LaneChanged input; LaneChangeCmd output

== matlab function speedgoat_target_model_2021b/Planning and Control/Subsystem3/Subsystem2/MATLAB Function ==
  data: u input; accel output; decel output
function [accel, decel] = fcn(u)
if(u>0)
    accel=u; decel=0;
elseif(u<0)
    accel=0; decel=-u;
else
    accel=0;decel=0;
end

== matlab function speedgoat_target_model_2021b/Planning and Control/MATLAB Function2 ==
  data: v input; RefVelCmd output; curvature input
function RefVelCmd = fcn(v,curvature)

    if abs(curvature) >= 0 && abs(curvature) <= 1e-2
        RefVelCmd = v;
    else
        r = 1/abs(curvature);
        RefVelCmd = min(v,sqrt(9.81*r*.7));
    end

== matlab function speedgoat_target_model_2021b/Planning and Control/MATLAB Function ==
  data: Dest input; D2D output; CurrentPose input
function D2D = fcn(Dest, CurrentPose)
CurrentPose(2) = -CurrentPose(2);
D2D = norm(Dest - CurrentPose(1:2)');

== stateflow chart speedgoat_target_model_2021b/Planning and Control/Chart ==
  settings: updateMethod=DISCRETE
  state Stationary
    du:
    VelCmd = 0;
    CurrentVelCmd = VelCmd;
    Navi = 0;
    Trans = 0;
    StopSim = 0;
  state Navigation
    state RailCrossing
      state Approaching
        en:
        ACC = 1;
        Tgap = 0;
        Trans = 0;
      state Stop
        en:
        VelCmd = 0;
        ACC = 0;
        CurrentVelCmd = VelCmd;
      state ExitScene
        en:
        ExitFlag = 1;
      state Transition
        en:
        ACC = 1;
        Tgap = 1;
        Trans = 1;
        VelCmd = SceneSpeed;
        CurrentVelCmd = VelCmd;
      (default) -> Navigation.RailCrossing.Approaching
      Navigation.RailCrossing.Approaching -> Navigation.RailCrossing.Stop [order 1] : [D2S <= 4]
      Navigation.RailCrossing.Stop -> Navigation.RailCrossing.Transition : [RRCross == 0 && ObjectDist > 14]
      Navigation.RailCrossing.Approaching -> Navigation.RailCrossing.ExitScene [order 2] : [SceneID ~= 10]
      Navigation.RailCrossing.Transition -> Navigation.RailCrossing.ExitScene : [SceneID == 0]
    state RoundAbout
      state Approaching
        en:
        ACC = 1;
        Trans = 0;
        Tgap = 0;
      state Stop
        en:
        VelCmd = 0;
        ACC = 0;
        CurrentVelCmd = VelCmd;
      state ExitScene
        en:
        ExitFlag = 1;
      state Transition
        en:
        ACC = 1;
        Tgap = 1;
        Trans = 1;
        VelCmd = SceneSpeed;
        CurrentVelCmd = VelCmd;
      (default) -> Navigation.RoundAbout.Approaching
      Navigation.RoundAbout.Approaching -> Navigation.RoundAbout.Stop [order 1] : [D2S <= 4]
      Navigation.RoundAbout.Stop -> Navigation.RoundAbout.Transition : [Clear2Go == 1]
      Navigation.RoundAbout.Approaching -> Navigation.RoundAbout.ExitScene [order 2] : [SceneID ~= 9]
      Navigation.RoundAbout.Transition -> Navigation.RoundAbout.ExitScene : [SceneID == 0]
    state DestCheck
      en,du:
      % dest reached?
      (default) -> (junction 47)
      (junction 47) -> (junction 48) [order 1] : [D2D < 2]
      (junction 48) -> (junction 50) : {DestReached = 1;}
      (junction 47) -> (junction 49) [order 2] : {DestReached = 0;}
      (junction 50) -> (junction 49) : {StopSim = 1;}
      (junction 49) -> (junction 51)
    state TrafficLight
      state Stop
        en:
        %CurrentVelCmd = VelCmd;
        %du:
        %if D2S < 7
        VelCmd = 0;
        %end
      state Approaching
        en:
        Tgap = 0;
        Trans = 0;
        %if TLstate(1,4) == 1
        ACC = 1;
        %else
        % ACC = 0;
        %end
      state Transition
        en:
        Trans = 1;
        ACC = 1;
        Tgap = 1;
        VelCmd = SceneSpeed;
        CurrentVelCmd = VelCmd;
      state ExitScene
        en:
        ExitFlag = 1;
      (default) -> Navigation.TrafficLight.Approaching
      Navigation.TrafficLight.Approaching -> Navigation.TrafficLight.Stop [order 1] : [D2S <= 4 && TLstate(1,4) < 3]
      Navigation.TrafficLight.Transition -> Navigation.TrafficLight.Approaching [order 2] : [TLstate(1,4) == 1 ]
      Navigation.TrafficLight.Stop -> Navigation.TrafficLight.Transition : [TLstate(1,4) == 3]
      Navigation.TrafficLight.Approaching -> Navigation.TrafficLight.Transition [order 2] : [TLstate(1,4) == 3]
      Navigation.TrafficLight.Approaching -> Navigation.TrafficLight.ExitScene [order 3] : [SceneID ~= 8]
      Navigation.TrafficLight.Transition -> Navigation.TrafficLight.ExitScene [order 1] : [SceneID == 0]
    state SceneRecognition
      en :
      VelCmd = RoadSpeed;
      CurrentVelCmd = VelCmd;
      ExitFlag = 0;
    state Go
      en:
      VelCmd = RoadSpeed;
      CurrentVelCmd = VelCmd;
      Trans = 0;
      ExitFlag = 0;
      ACC = 0;
    state StopSign
      state Approaching
        en:
        ACC = 1;
        Trans = 0;
        Tgap = 0;
      state Stop
        en:
        VelCmd = 0;
        ACC = 0;
        CurrentVelCmd = VelCmd;
      state ExitScene
        en:
        ExitFlag = 1;
      state Transition
        en:
        Trans = 1;
        ACC = 0;
        Tgap = 1;
        VelCmd = SceneSpeed;
        CurrentVelCmd = VelCmd;
      (default) -> Navigation.StopSign.Approaching
      Navigation.StopSign.Approaching -> Navigation.StopSign.Stop [order 1] : [D2S <= 7]
      Navigation.StopSign.Stop -> Navigation.StopSign.Transition : [after(3,sec) && Clear2Go == 1]
      Navigation.StopSign.Approaching -> Navigation.StopSign.ExitScene [order 2] : [SceneID ~= 7]
      Navigation.StopSign.Transition -> Navigation.StopSign.ExitScene : [SceneID == 0]
    Go -> RailCrossing [order 2] : [SceneID == 10]
    SceneRecognition -> RailCrossing [order 1] : [SceneID == 10]
    RailCrossing -> Go : [ExitFlag == 1]
    Go -> RoundAbout [order 4] : [SceneID == 9]
    SceneRecognition -> RoundAbout [order 2] : [SceneID == 9]
    RoundAbout -> Go : [ExitFlag == 1]
    (default) -> DestCheck
    SceneRecognition -> TrafficLight [order 4] : [SceneID == 8]
    DestCheck -> SceneRecognition : [DestReached == 0]
    Go -> TrafficLight [order 3] : [SceneID == 8]
    SceneRecognition -> DestCheck [order 5] : [D2D < 2]
    SceneRecognition -> StopSign [order 3] : [SceneID == 7]
    TrafficLight -> Go : [ExitFlag == 1]
    StopSign -> Go : [ExitFlag == 1]
    Go -> DestCheck [order 1] : [SceneID == 0]
    Go -> StopSign [order 5] : [SceneID == 7]
  (default) -> Stationary
  Stationary -> Navigation : [Navigate == 1]
  Navigation -> Stationary : [Navigate == 0 || DestReached == 1]
  data: TLstate input; ApproachingSpeed input; ObjectDist input; SceneSpeed input; SDist input; RRCross input; D2S input; DestReached local; Navigate input; ExitFlag local; D2D input; Clear2Go input; RoadSpeed input; CurrentVelCmd local; Navi local; VelCmd output; SceneID input; ACC output; Tgap output; Trans output; StopSim output
